simulink subsystem "error_check_sub"  (R2022b)
settings: Solver=VariableStepAuto  StartTime=0.0  StopTime=10.0  RelTol=1e-3
settings Model: Creator=Edp  LastModifiedBy=Edp

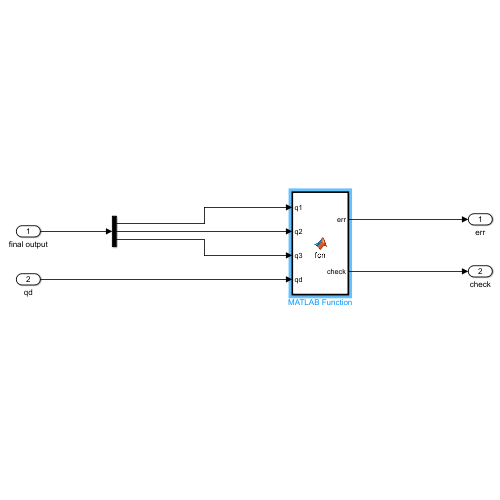
[thumbnail: Simulink's stored preview of the top-level diagram]
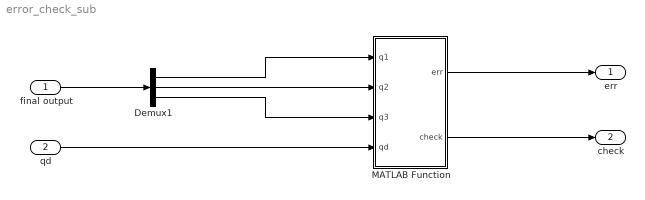
== system error_check_sub ==
  final output : Inport
  qd : Inport  Port=2
  Demux1 : Demux  Outputs=3
  MATLAB Function : MATLAB Function  TreatAsAtomicUnit=on  SystemSampleTime=0.1
  err : Outport
  check : Outport  Port=2
  wires:
  MATLAB Function/1(err) -> err/1
  Demux1/1 -> MATLAB Function/1(q1)
  final output/1 -> Demux1/1
  MATLAB Function/2(check) -> check/1
  Demux1/2 -> MATLAB Function/2(q2)
  Demux1/3 -> MATLAB Function/3(q3)
  qd/1 -> MATLAB Function/4(qd)

== matlab function error_check_sub/MATLAB Function ==
  settings: updateMethod=DISCRETE
  data: q1 input; q2 input; q3 input; qd input; err output; check output
function [err, check] = fcn(q1,q2,q3,qd)
check = 0;
thresh = 1;
err = [10, 10, 10];
qq1 = [q1(1) q1(2)];
qq2 = [q2(1) q2(2)];
qq3 = [q3(1) q3(2)];
qqd = [qd(1) qd(2)];

err(1) = norm(qqd - qq1);
err(2) = norm(qqd - qq2);
err(3) = norm(qqd - qq3);

persistent k;
if isempty(k)
    k = 0;
else
    if err(1) < thresh && err(2) < thresh && err(3) < thresh
        k = k + 1;
    else
        k = 0;
        check = 0;
    end
        
    if k > 15
        check = 1;
    end
end
